simulink model "th4_general"  (R2023b)
settings: Solver=VariableStepAuto  StartTime=0.0  StopTime=1000  RelTol=1e-3
values from neighbouring files (symbols this model uses):
  A = 1.2    [part1_q4.m]
  battery_capacity = 20    [th4_init.m]
  Cd = 0.5    [part1_q4.m]
  f = 0.015    [part1_q4.m]    (also in th4_q19.m; th4_q19_claude.m)
  g = 9.81    [part1_q4.m]    (also in th4_q19.m; th4_q19_claude.m; th4_q19_create_road_grade.m = segments(i,3))
  m = 1250    [part1_q4.m]    (also in th4_q19_battery_pps.m = 1305.3)
  m_eqv = m + I_w_total/r^2 + I_e*(G*R)^2/r^2    (= 1305.28194444)    [part1_q4.m]    (also in th4_q19.m = 1305.3; th4_q19_claude.m = 1305.3)
  mu_driveline = 0.8    [th4_init.m]
  mu_generator = 0.9    [th4_init.m]
  R_w = 0.5    [th4_init.m]
  ro = 1.225    [part1_q4.m]
  SOC_init = 0.6    [th4_init.m]
  SOC_max = 0.95    [th4_init.m]
  SOC_min = 0.2    [th4_init.m]
libraries: simulink x2, simulink_extras x2, slpidlib x1
settings Model: Creator=yusufcagriogut  LastModifiedBy=yusufcagriogut

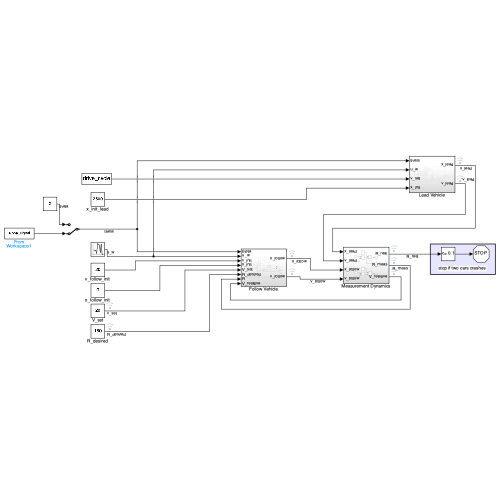
[thumbnail: Simulink's stored preview of the top-level diagram]
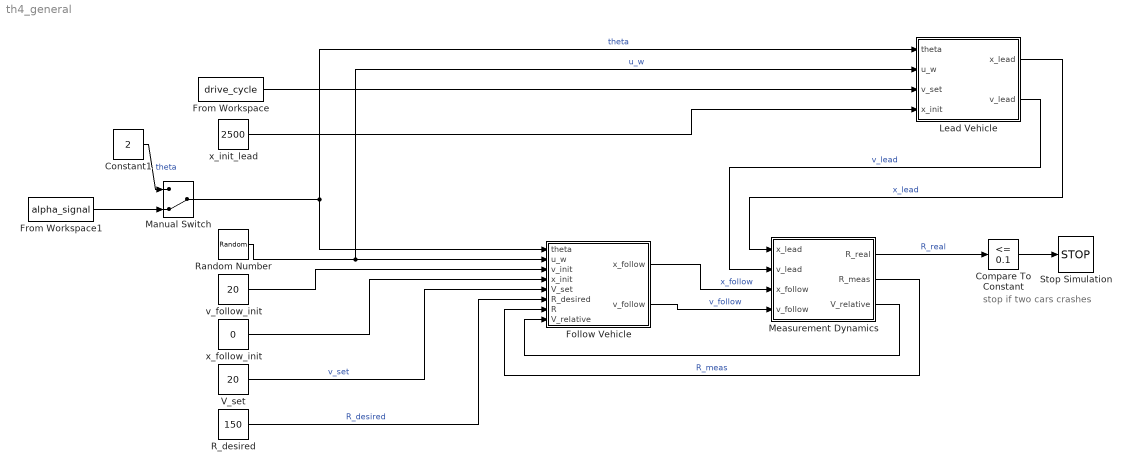
== system th4_general ==
  note: stop if two cars crashes
  Compare To Constant : simulink/Logic and Bit Operations/Compare To Constant  relop=<=  const=0.1  OutDataTypeStr=boolean
  Constant1 : Constant  Value=2
  Follow Vehicle : Subsystem
  From Workspace : FromWorkspace  VariableName=drive_cycle
  From Workspace1 : FromWorkspace  VariableName=alpha_signal
  Lead Vehicle : Subsystem
  Manual Switch : ManualSwitch  CurrentSetting=0
  Measurement Dynamics : Subsystem
  R_desired : Constant  Value=150
  Random Number : RandomNumber  Variance=2  SampleTime=2
  Stop Simulation : Stop
  V_set : Constant  Value=20
  v_follow_init : Constant  Value=20
  x_follow_init : Constant  Value=0
  x_init_lead : Constant  Value=2500
  wires:
  Lead Vehicle/2(v_lead) -> Measurement Dynamics/2(v_lead)  "v_lead"
  Lead Vehicle/1(x_lead) -> Measurement Dynamics/1(x_lead)  "x_lead"
  Measurement Dynamics/2(R_meas) -> Follow Vehicle/7(R)  "R_meas"
  Follow Vehicle/1(x_follow) -> Measurement Dynamics/3(x_follow)  "x_follow"
  Follow Vehicle/2(v_follow) -> Measurement Dynamics/4(v_follow)  "v_follow"
  Measurement Dynamics/3(V_relative) -> Follow Vehicle/8(V_relative)
  Manual Switch/1 -> Follow Vehicle/1(theta), Lead Vehicle/1(theta)  "theta"
  Random Number/1 -> Lead Vehicle/2(u_w), Follow Vehicle/2(u_w)  "u_w"
  From Workspace/1 -> Lead Vehicle/3(v_set)
  x_init_lead/1 -> Lead Vehicle/4(x_init)
  v_follow_init/1 -> Follow Vehicle/3(v_init)
  x_follow_init/1 -> Follow Vehicle/4(x_init)
  Measurement Dynamics/1(R_real) -> Compare To Constant/1  "R_real"
  V_set/1 -> Follow Vehicle/5(V_set)  "v_set"
  R_desired/1 -> Follow Vehicle/6(R_desired)  "R_desired"
  Compare To Constant/1 -> Stop Simulation/1
  Constant1/1 -> Manual Switch/1  "theta"
  From Workspace1/1 -> Manual Switch/2

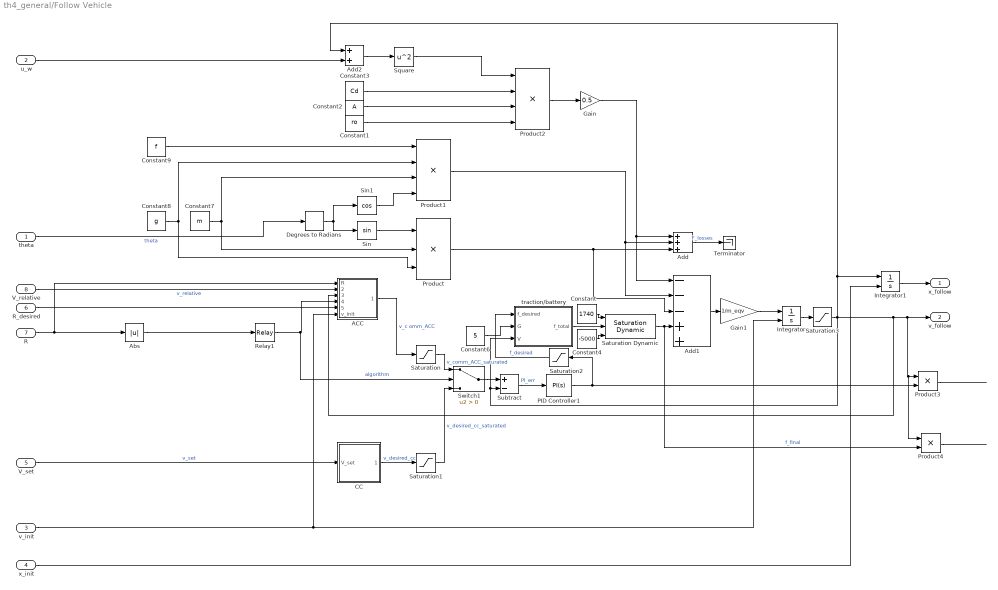
== system th4_general/Follow Vehicle ==
  theta : Inport
  u_w : Inport  Port=2
  v_init : Inport  Port=3
  x_init : Inport  Port=4
  V_set : Inport  Port=5
  R_desired : Inport  Port=6
  R : Inport  Port=7
  V_relative : Inport  Port=8
  ACC : Subsystem
  Abs : Abs  SaturateOnIntegerOverflow=off
  Add : Sum  Inputs=+++
  Add1 : Sum  Inputs=---++
  Add2 : Sum
  CC : Subsystem
  Constant : Constant  Value=1740
  Constant1 : Constant  Value=ro
  Constant2 : Constant  Value=A
  Constant3 : Constant  Value=Cd
  Constant4 : Constant  Value=-5000
  Constant6 : Constant  Value=5
  Constant7 : Constant  Value=m
  Constant8 : Constant  Value=g
  Constant9 : Constant  Value=f
  Degrees to Radians : simulink_extras/Transformations/Degrees to Radians
  Gain : Gain  Gain=0.5
  Gain1 : Gain  Gain=1/m_eqv
  Integrator : Integrator  InitialConditionSource=external  InitialCondition=33
  Integrator1 : Integrator  InitialConditionSource=external
  PID Controller1 : slpidlib/PID Controller  Controller=PI  Form=Parallel  TimeDomain=Continuous-time  UseExternalTs=off  SampleTime=-1  IntegratorMethod=Forward Euler  FilterMethod=Forward Euler  ControllerParametersSource=internal  P=600  I=50  UseKiTs=off  D=0  N=12.815158437423  UseFilter=on  TunerSelectOption=Transfer Function Based (PID Tuner App)  InitialConditionSource=internal  InitialConditionForIntegrator=0  InitialConditionForFilter=0  DifferentiatorICPrevScaledInput=0  ExternalReset=none  TrackingMode=off  Kt=1  LimitOutput=off  SatLimitsSource=internal  UpperSaturationLimit=inf  LowerSaturationLimit=-inf  LinearizeAsGain=on  AntiWindupMode=none  Kb=1  LimitIntegrator=off  UpperIntegratorSaturationLimit=inf  LowerIntegratorSaturationLimit=-inf  POutMin=[]  POutMax=[]  IOutMin=[]  IOutMax=[]  DOutMin=[]  DOutMax=[]  NOutMin=[]  NOutMax=[]  SumOutMin=[]  SumOutMax=[]  SaturationOutMin=[]  SaturationOutMax=[]  PParamMin=[]  PParamMax=[]  IParamMin=[]  IParamMax=[]  DParamMin=[]  DParamMax=[]  NParamMin=[]  NParamMax=[]  KbParamMin=[]  KbParamMax=[]  KtParamMin=[]  KtParamMax=[]  KbOutMin=[]  KbOutMax=[]  KtOutMin=[]  KtOutMax=[]  IntegratorOutMin=[]  IntegratorOutMax=[]  FilterOutMin=[]  FilterOutMax=[]  SumI1OutMin=[]  SumI1OutMax=[]  SumI2OutMin=[]  SumI2OutMax=[]  SumI3OutMin=[]  SumI3OutMax=[]  SumI4OutMin=[]  SumI4OutMax=[]  SumDOutMin=[]  SumDOutMax=[]  DifferentiatorOutMin=[]  DifferentiatorOutMax=[]  FilterDiffOutCoefMin=[]  FilterDiffOutCoefMax=[]  ReciprocalOutMin=[]  ReciprocalOutMax=[]  SumDenOutMin=[]  SumDenOutMax=[]  SumNumOutMin=[]  SumNumOutMax=[]  DivideOutMin=[]  DivideOutMax=[]  UdiffTsProdOutMin=[]  UdiffTsProdOutMax=[]  NTsProdOutMin=[]  NTsProdOutMax=[]  UintegralTsProdOutMin=[]  UintegralTsProdOutMax=[]  UngainTsProdOutMin=[]  UngainTsProdOutMax=[]  ClampingZeroOutDataTypeStr=Inherit: Inherit via back propagation  ClampingZeroOutMin=[]  ClampingZeroOutMax=[]  FilterDenConstantOutDataTypeStr=Inherit: Inherit via back propagation  FilterDenConstantOutMin=[]  FilterDenConstantOutMax=[]  PCopyOutDataTypeStr=Inherit: Inherit via back propagation  PCopyOutMin=[]  PCopyOutMax=[]  NCopyOutDataTypeStr=Inherit: Inherit via back propagation  NCopyOutMin=[]  NCopyOutMax=[]  IntegratorContinuousStateAttributes=''  IntegratorStateMustResolveToSignalObject=off  IntegratorRTWStateStorageClass=Auto  FilterContinuousStateAttributes=''  FilterStateMustResolveToSignalObject=off  FilterRTWStateStorageClass=Auto  ParallelPVariant=InternalParameters  IdealPVariant=Disabled  IVariant=InternalParameters  DVariant=Disabled  IntegratorVariant=Continuous  SatVariant=Disabled  AWVariant=Passthrough  PCopyVariant=Disabled  TRVariant=Disabled  FdbkBlocksVariant=Forward  IdealPFdbkVariant=Disabled  SatFdbkVariant=Disabled  DerivativeFilterVariant=Disabled  NVariant=Disabled  NCopyVariant=Disabled_SignalSpec  FilterICVariant=Disabled  IntegratorICVariant=InternalICs  ExternalResetVariant=Disabled  TRSumVariant=Passthrough  SumFdbkVariant=Disabled  SumVariant=Sum_PI  TsampFilterVariant=InternalTs  TsampNgainVariant=Passthrough  TsampIntegralVariant=Disabled_SignalSpec  ExternalSaturationOutDataTypeStr=Inherit: Same as second input
  Product : Product  Inputs=3
  Product1 : Product  Inputs=4
  Product2 : Product  Inputs=4
  Product3 : Product
  Product4 : Product
  Relay1 : Relay  OnSwitchValue=160  OffSwitchValue=140  OnOutputValue=0  OffOutputValue=1
  Saturation : Saturate  UpperLimit=50  LowerLimit=-50
  Saturation Dynamic : simulink/Discontinuities/Saturation Dynamic  OutMin=[]  OutMax=[]  OutDataTypeStr=Inherit: Same as second input  OutDataType=fixdt(1, 16)  OutScaling=2^-10  DoSatur=off
  Saturation1 : Saturate  UpperLimit=50  LowerLimit=0
  Saturation2 : Saturate  UpperLimit=1740  LowerLimit=-5000
  Saturation3 : Saturate  UpperLimit=120  LowerLimit=0
  Sin : Trigonometry
  Sin1 : Trigonometry  Operator=cos
  Square : Math  Operator=square
  Subtract : Sum  Inputs=+-
  Switch1 : Switch  Criteria=u2 > Threshold  SaturateOnIntegerOverflow=off  InputSameDT=off
  Terminator : Terminator
  traction/battery : Subsystem
  x_follow : Outport
  v_follow : Outport  Port=2
  wires:
  Integrator1/1 -> x_follow/1
  R/1 -> ACC/1(R), Abs/1
  Abs/1 -> Relay1/1
  Gain1/1 -> Integrator/1
  Add1/1 -> Gain1/1
  Product2/1 -> Gain/1
  Add2/1 -> Square/1
  Constant1/1 -> Product2/4
  Constant2/1 -> Product2/3
  Constant3/1 -> Product2/2
  u_w/1 -> Add2/2
  Square/1 -> Product2/1
  Integrator/1 -> Saturation3/1
  Gain/1 -> Add/1, Add1/1
  theta/1 -> Degrees to Radians/1  "theta"
  Sin/1 -> Product/1
  Product/1 -> Add1/3, Add/3
  Constant8/1 -> Product/3, Product1/2
  Sin1/1 -> Product1/4
  Constant7/1 -> Product/2, Product1/3
  Product1/1 -> Add1/2, Add/2
  Constant9/1 -> Product1/1
  Degrees to Radians/1 -> Sin/1, Sin1/1
  v_init/1 -> ACC/6(v_init), Integrator/2
  x_init/1 -> Integrator1/2
  V_relative/1 -> ACC/2(V_relative)  "v_relative"
  V_set/1 -> CC/1(V_set)  "v_set"
  Saturation/1 -> Switch1/1  "v_comm_ACC_saturated"
  ACC/1(v_desired) -> Saturation/1  "v_c omm_ACC"
  Switch1/1 -> Subtract/1
  CC/1(V_desired) -> Saturation1/1  "v_desired_cc"
  Saturation1/1 -> Switch1/3  "v_desired_cc_saturated"
  R_desired/1 -> ACC/5(R_desired)
  Saturation Dynamic/1 -> Product4/2, Add1/4  "f_final"
  Constant/1 -> Saturation Dynamic/1
  Constant4/1 -> Saturation Dynamic/3
  PID Controller1/1 -> Saturation2/1, Product3/2
  Subtract/1 -> PID Controller1/1  "PI_err"
  Relay1/1 -> ACC/4(active), Switch1/2  "algorithm"
  Product3/1 -> ?
  Product4/1 -> ?
  Constant6/1 -> traction/battery/2(G)
  Saturation2/1 -> traction/battery/1(f_desired)  "f_desired"
  Saturation3/1 -> Add2/1, Integrator1/1, traction/battery/3(V), Subtract/2, ACC/3(V_follow), Product4/1, Product3/1, v_follow/1
  traction/battery/1(f_total) -> Saturation Dynamic/2
  Add/1 -> Terminator/1  "F_losses"

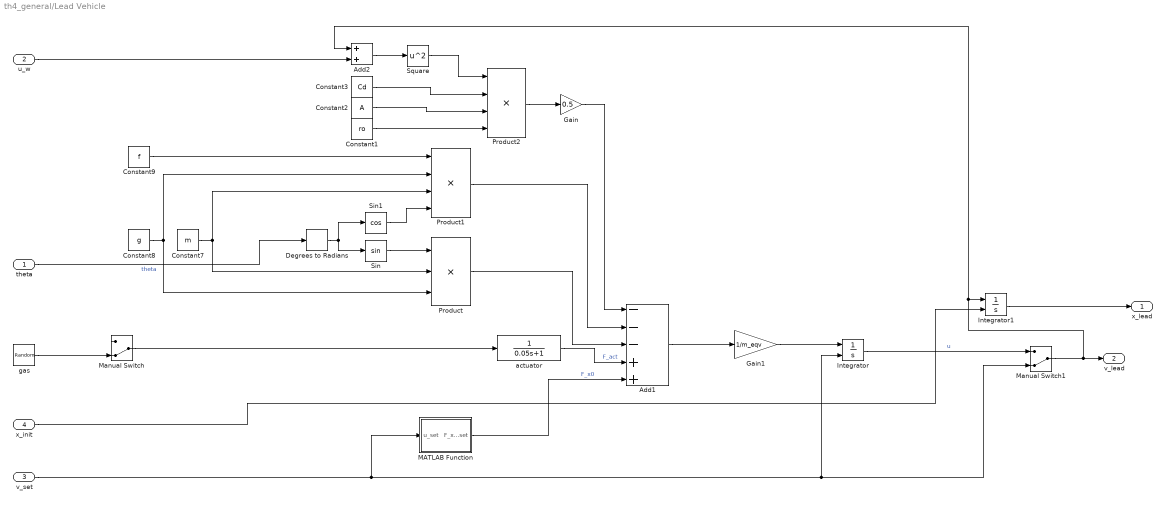
== system th4_general/Lead Vehicle ==
  theta : Inport
  u_w : Inport  Port=2
  v_set : Inport  Port=3
  x_init : Inport  Port=4
  Add1 : Sum  Inputs=---++
  Add2 : Sum
  Constant1 : Constant  Value=ro
  Constant2 : Constant  Value=A
  Constant3 : Constant  Value=Cd
  Constant7 : Constant  Value=m
  Constant8 : Constant  Value=g
  Constant9 : Constant  Value=f
  Degrees to Radians : simulink_extras/Transformations/Degrees to Radians
  Gain : Gain  Gain=0.5
  Gain1 : Gain  Gain=1/m_eqv
  Integrator : Integrator  InitialConditionSource=external  InitialCondition=33
  Integrator1 : Integrator  InitialConditionSource=external
  MATLAB Function : MATLAB Function  TreatAsAtomicUnit=on
  Manual Switch : ManualSwitch  CurrentSetting=0
  Manual Switch1 : ManualSwitch  CurrentSetting=0
  Product : Product  Inputs=3
  Product1 : Product  Inputs=4
  Product2 : Product  Inputs=4
  Sin : Trigonometry
  Sin1 : Trigonometry  Operator=cos
  Square : Math  Operator=square
  actuator : TransferFcn  Denominator=[0.05 1]
  gas : RandomNumber  Variance=0  SampleTime=2
  x_lead : Outport
  v_lead : Outport  Port=2
  wires:
  Integrator1/1 -> x_lead/1
  Gain1/1 -> Integrator/1
  Add1/1 -> Gain1/1
  v_set/1 -> Manual Switch1/2, Integrator/2, MATLAB Function/1(u_set)
  actuator/1 -> Add1/4  "F_act"
  Product2/1 -> Gain/1
  Add2/1 -> Square/1
  Constant1/1 -> Product2/4
  Constant2/1 -> Product2/3
  Constant3/1 -> Product2/2
  u_w/1 -> Add2/2
  Square/1 -> Product2/1
  Integrator/1 -> Manual Switch1/1  "u"
  Gain/1 -> Add1/1
  theta/1 -> Degrees to Radians/1  "theta"
  Sin/1 -> Product/1
  Product/1 -> Add1/3
  Constant8/1 -> Product/3, Product1/2
  Sin1/1 -> Product1/4
  Constant7/1 -> Product/2, Product1/3
  Product1/1 -> Add1/2
  Constant9/1 -> Product1/1
  Degrees to Radians/1 -> Sin/1, Sin1/1
  x_init/1 -> Integrator1/2
  MATLAB Function/1(F_x0_set) -> Add1/5  "F_x0"
  Manual Switch/1 -> actuator/1
  gas/1 -> Manual Switch/2
  Manual Switch1/1 -> Add2/1, Integrator1/1, v_lead/1

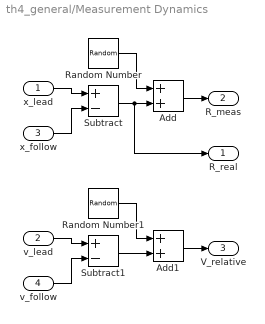
== system th4_general/Measurement Dynamics ==
  x_lead : Inport
  v_lead : Inport  Port=2
  x_follow : Inport  Port=3
  v_follow : Inport  Port=4
  Add : Sum
  Add1 : Sum
  Random Number : RandomNumber  Variance=0.2  SampleTime=0.1
  Random Number1 : RandomNumber  Variance=0.1  SampleTime=0.1
  Subtract : Sum  Inputs=+-
  Subtract1 : Sum  Inputs=+-
  R_real : Outport
  R_meas : Outport  Port=2
  V_relative : Outport  Port=3
  wires:
  Add/1 -> R_meas/1
  x_lead/1 -> Subtract/1
  x_follow/1 -> Subtract/2
  Subtract/1 -> R_real/1, Add/2
  Random Number/1 -> Add/1
  Add1/1 -> V_relative/1
  Subtract1/1 -> Add1/2
  Random Number1/1 -> Add1/1
  v_follow/1 -> Subtract1/2
  v_lead/1 -> Subtract1/1

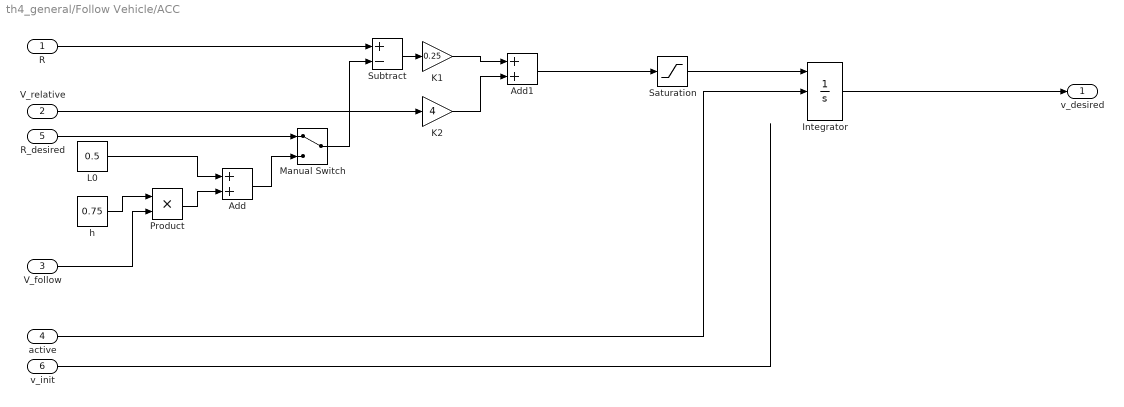
== system th4_general/Follow Vehicle/ACC ==
  R : Inport
  V_relative : Inport  Port=2
  V_follow : Inport  Port=3
  active : Inport  Port=4
  R_desired : Inport  Port=5
  v_init : Inport  Port=6
  Add : Sum
  Add1 : Sum
  Integrator : Integrator  ExternalReset=rising  InitialConditionSource=external  LimitOutput=on  UpperSaturationLimit=50  LowerSaturationLimit=0
  K1 : Gain  Gain=0.25
  K2 : Gain  Gain=4
  L0 : Constant  Value=0.5
  Manual Switch : ManualSwitch
  Product : Product
  Saturation : Saturate  UpperLimit=2.5  LowerLimit=-1
  Subtract : Sum  Inputs=+-
  h : Constant  Value=0.75
  v_desired : Outport
  wires:
  R/1 -> Subtract/1
  h/1 -> Product/1
  V_follow/1 -> Product/2
  L0/1 -> Add/1
  Product/1 -> Add/2
  Subtract/1 -> K1/1
  V_relative/1 -> K2/1
  K1/1 -> Add1/1
  Add1/1 -> Saturation/1
  active/1 -> Integrator/2
  R_desired/1 -> Manual Switch/1
  K2/1 -> Add1/2
  v_init/1 -> ?
  Add/1 -> Manual Switch/2
  Manual Switch/1 -> Subtract/2
  Saturation/1 -> Integrator/1
  Integrator/1 -> v_desired/1

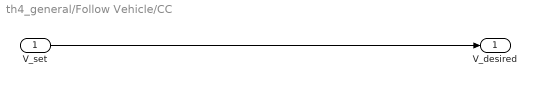
== system th4_general/Follow Vehicle/CC ==
  V_set : Inport
  V_desired : Outport
  wires:
  V_set/1 -> V_desired/1

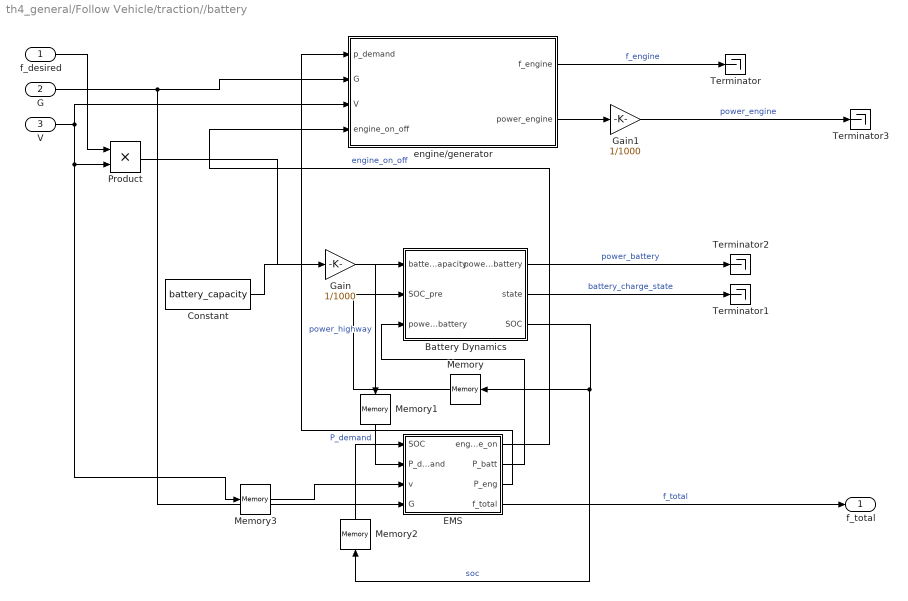
== system th4_general/Follow Vehicle/traction//battery ==
  f_desired : Inport
  G : Inport  Port=2
  V : Inport  Port=3
  Battery Dynamics : MATLAB Function  TreatAsAtomicUnit=on
  Constant : Constant  Value=battery_capacity
  EMS : Subsystem
  Gain : Gain  Gain=1/1000
  Gain1 : Gain  Gain=1/1000
  Memory : Memory  InitialCondition=SOC_init
  Memory1 : Memory
  Memory2 : Memory  InitialCondition=SOC_init
  Memory3 : Memory  InitialCondition=20
  Product : Product
  Terminator{,1..3} (4 alike) : Terminator
  engine/generator : Subsystem
  f_total : Outport
  wires:
  f_desired/1 -> Product/1
  G/1 -> engine/generator/2(G), EMS/4(G)
  V/1 -> Memory3/1, Product/2, engine/generator/3(V)
  engine/generator/2(power_engine) -> Gain1/1
  Battery Dynamics/3(SOC) -> Memory2/1, Memory/1  "soc"
  Product/1 -> Gain/1
  Memory/1 -> Battery Dynamics/2(SOC_pre)
  Constant/1 -> Battery Dynamics/1(battery_capacity)
  engine/generator/1(f_engine) -> Terminator/1  "f_engine"
  Battery Dynamics/2(state) -> Terminator1/1  "battery_charge_state"
  Battery Dynamics/1(power_battery) -> Terminator2/1  "power_battery"
  Gain/1 -> Memory1/1  "power_highway"
  Gain1/1 -> Terminator3/1  "power_engine"
  EMS/1(engine_on) -> engine/generator/4(engine_on_off)  "engine_on_off"
  EMS/3(P_eng) -> engine/generator/1(p_demand)
  EMS/2(P_batt) -> Battery Dynamics/3("power_battery ")
  Memory1/1 -> EMS/2(P_demand)  "P_demand"
  Memory2/1 -> EMS/1(SOC)
  Memory3/1 -> EMS/3(v)
  EMS/4(f_total) -> f_total/1  "f_total"

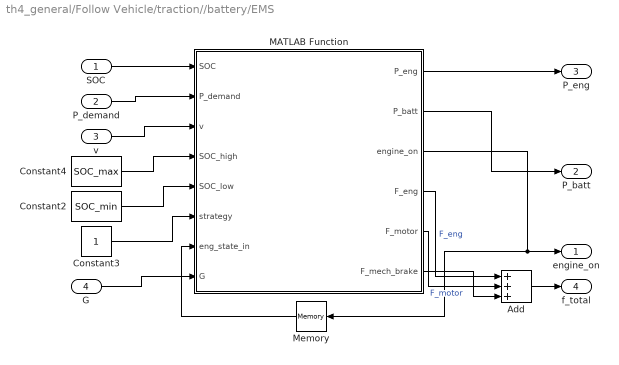
== system th4_general/Follow Vehicle/traction//battery/EMS ==
  SOC : Inport
  P_demand : Inport  Port=2
  v : Inport  Port=3
  G : Inport  Port=4
  Add : Sum  Inputs=+++
  Constant2 : Constant  Value=SOC_min
  Constant3 : Constant
  Constant4 : Constant  Value=SOC_max
  MATLAB Function : MATLAB Function  TreatAsAtomicUnit=on
  Memory : Memory  InitialCondition=1
  engine_on : Outport
  P_batt : Outport  Port=2
  P_eng : Outport  Port=3
  f_total : Outport  Port=4
  wires:
  Constant3/1 -> MATLAB Function/6(strategy)
  SOC/1 -> MATLAB Function/1(SOC)
  Constant2/1 -> MATLAB Function/5(SOC_low)
  Constant4/1 -> MATLAB Function/4(SOC_high)
  P_demand/1 -> MATLAB Function/2(P_demand)
  v/1 -> MATLAB Function/3(v)
  MATLAB Function/2(P_batt) -> P_batt/1
  MATLAB Function/1(P_eng) -> P_eng/1
  MATLAB Function/3(engine_on) -> Memory/1, engine_on/1
  Memory/1 -> MATLAB Function/7(eng_state_in)
  G/1 -> MATLAB Function/8(G)
  MATLAB Function/4(F_eng) -> Add/1  "F_eng"
  MATLAB Function/5(F_motor) -> Add/2  "F_motor"
  Add/1 -> f_total/1
  MATLAB Function/6(F_mech_brake) -> Add/3

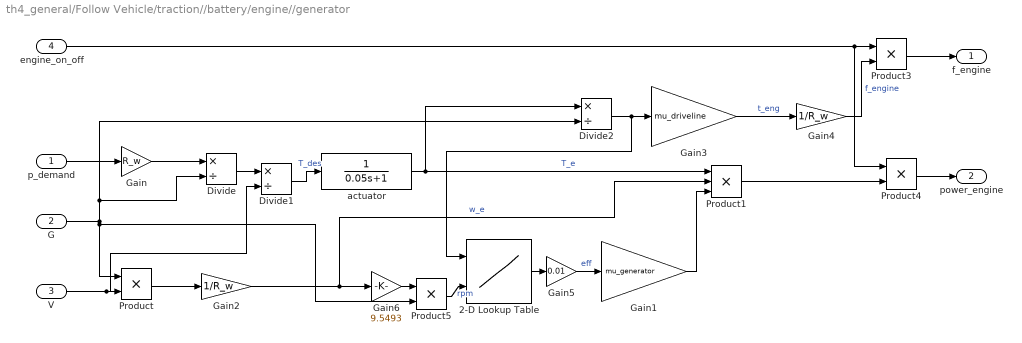
== system th4_general/Follow Vehicle/traction//battery/engine//generator ==
  p_demand : Inport
  G : Inport  Port=2
  V : Inport  Port=3
  engine_on_off : Inport  Port=4
  2-D Lookup Table : Lookup_n-D  BreakpointsForDimension1=[0, 20, 40, 60, 80, 100, 120, 140, 160, 174]  BreakpointsForDimension2=[800, 1200, 1600, 2000, 2500, 3000, 3500, 4000, 4500, 5000, 5500, 6000]  Table=[3,4,5,5.50000000000000,6,6,5.50000000000000,5,4.50000000000000,4,3.50000000000000,3;8,11,14,16,17,17.5000000000000,17,16,15,13.5000000000000,11.5000000000000,9;13,18,22,25,27,28,27.5000000000000,26.5000000000000,25,22.5000000000000,19.5000000000000,15;17,22,27,30,32,33,32.5000000000000,31.5000000000000,30,27.5000000000000,24,19;20,26,30.5000000000000,33.5000000000000,35,35.5000000000000,35,34,32.5000000000000,30,26.5000000000000,21.5000000000000;22.5000000000000,28.5000000000000,32.5000000000000,35,36.5000000000000,37,36.5000000000000,35.5000000000000,34,31.5000000000000,28,23;24,30,33.5000000000000,35.5000000000000,37,37.5000000000000,37,36,34.5000000000000,32,28.5000000000000,23.5000000000000;24.5000000000000,30.5000000000000,34,36,37.5000000000000,38,37.5000000000000,36.5000000000000,35,32.5000000000000,29,24;24,30,33.5000000000000,36,37.5000000000000,38,37.5000000000000,36.5000000000000,35,32.5000000000000,29,24;23,29.5000000000000,33,35.5000000000000,37,37.5000000000000,37,36,34.5000000000000,32,28.5000000000000,23.5000000000000]  InternalRulePriority=Speed  RndMeth=Simplest
      settings: InputPortMap=u0,u1
  Divide : Product  Inputs=*/
  Divide1 : Product  Inputs=*/
  Divide2 : Product  Inputs=*/
  Gain : Gain  Gain=R_w
  Gain1 : Gain  Gain=mu_generator
  Gain2 : Gain  Gain=1/R_w
  Gain3 : Gain  Gain=mu_driveline
  Gain4 : Gain  Gain=1/R_w
  Gain5 : Gain  Gain=0.01
  Gain6 : Gain  Gain=9.5493
  Product{,3..5} (4 alike) : Product
  Product1 : Product  Inputs=3
  actuator : TransferFcn  Denominator=[0.05 1]
  f_engine : Outport
  power_engine : Outport  Port=2
  wires:
  Gain4/1 -> Product3/2  "f_engine"
  Divide2/1 -> 2-D Lookup Table/1, Gain3/1
  Gain/1 -> Divide/1
  Gain3/1 -> Gain4/1  "t_eng"
  p_demand/1 -> Gain/1
  Product/1 -> Gain2/1
  2-D Lookup Table/1 -> Gain5/1
  G/1 -> Product5/2, Product/1, Divide2/2, Divide/2
  Divide/1 -> Divide1/1
  actuator/1 -> Divide2/1, Product1/1  "T_e"
  V/1 -> Divide1/2, Product/2
  Gain2/1 -> Gain6/1, Product1/2  "w_e"
  Gain5/1 -> Gain1/1  "eff"
  Gain6/1 -> Product5/1
  engine_on_off/1 -> Product4/1, Product3/1
  Product3/1 -> f_engine/1
  Product1/1 -> Product4/2
  Product4/1 -> power_engine/1
  Divide1/1 -> actuator/1  "T_des"
  Product5/1 -> 2-D Lookup Table/2  "rpm"
  Gain1/1 -> Product1/3

== matlab function th4_general/Lead Vehicle/MATLAB Function ==
  data: u_set input; F_x0_set output
function F_x0_set = fcn(u_set)
m = 1250;
ro = 1.225;
A = 1.2;
Cd = 0.5;
f = 0.015;
R = 3;
I_e = 0.15;
r = 0.3;
I_w = 1.0;
u_0 = 40;
u_w = 2;
g = 9.81;
theta_0 = 0;
F_x0_set = m*g*sin(theta_0) + f*m*g*cos(theta_0) + ...
    0.5*ro*A*Cd*(u_set+u_w)^2;
end

== matlab function th4_general/Follow Vehicle/traction//battery/Battery Dynamics ==
  data: power_battery output; battery_capacity input; SOC_pre input; state output; SOC output; power_battery input
function [power_battery, state,SOC] = fcn(battery_capacity, SOC_pre, power_battery)
if power_battery>0
    state = 0; % supply
else
    state = 1; % charging
end
SOC = SOC_pre - power_battery * 1 / 3600 / 0.92 / battery_capacity;
if SOC<0
    SOC = 0;
elseif SOC>1
    SOC = 1;
end
end

== matlab function th4_general/Follow Vehicle/traction//battery/EMS/MATLAB Function ==
  data: SOC input; P_eng output; P_demand input; v input; SOC_high input; SOC_low input; strategy input; P_batt output; engine_on output; eng_state_in input; G input; F_eng output; F_motor output; F_mech_brake output
function [P_eng, P_batt, engine_on, F_eng, F_motor,F_mech_brake] = EMS(SOC, P_demand, v, SOC_high, SOC_low, strategy, eng_state_in, G)

%% Parameters
P_eng_max   = 60.0;
P_eng_opt   = 20.0;
v_min       = 1.0;
P_regen_max = 30.0;
r_wheel     = 0.5;
T_eng_max   = 174;
P_motor_kW  = 69.0;
Vb          = 40/3.6;
F_motor_max = (P_motor_kW * 1000) / Vb;

%% Defaults
P_eng     = 0;
P_batt    = 0;
engine_on = 0;
P_mech_brake = 0;
%% ---- Decision logic (no early returns) ----
if P_demand < 0
    if SOC >= SOC_high
        P_batt       = 0;
        P_mech_brake = P_demand;        % all braking is mechanical
    else
        P_batt       = max(P_demand, -P_regen_max);
        P_mech_brake = P_demand - P_batt;  % remainder after regen
    end
    P_eng     = 0;
    engine_on = 0;

elseif v < v_min
    %% Standstill
    P_eng     = 0;
    P_batt    = P_demand;
    engine_on = 0;

elseif strategy == 1
    %% On-Off
    if SOC <= SOC_low
        P_eng     = min(P_eng_opt, P_eng_max);
        P_batt    = P_demand - P_eng;
        engine_on = 1;
    elseif SOC >= SOC_high
        P_eng     = 0;
        P_batt    = P_demand;
        engine_on = 0;
    else
        if eng_state_in == 1
            P_eng  = min(P_eng_opt, P_eng_max);
            P_batt = P_demand - P_eng;
        else
            P_eng  = 0;
            P_batt = P_demand;
        end
        engine_on = eng_state_in;
    end

elseif strategy == 2
    %% Max SOC
    if SOC >= SOC_high
        % Battery full — engine covers only exact demand
        P_eng     = min(P_demand, P_eng_max);
        P_batt    = P_demand - P_eng;
        engine_on = 1;

    elseif SOC < SOC_low
        % Battery critically low — engine at max to recharge fast
        P_eng     = P_eng_max;
        P_batt    = P_demand - P_eng;
        engine_on = 1;

    else
        % Normal band — engine ALWAYS runs at optimal point
        % regardless of P_demand, to proactively charge battery
        P_eng     = P_eng_opt;           % <-- was: min(P_demand, P_eng_opt)
        P_batt    = P_demand - P_eng;    % will be negative = charging
        engine_on = 1;                   % <-- was: conditional on P_eng > 0
    end

else
    P_eng     = 0;
    P_batt    = P_demand;
    engine_on = 0;
end

%% ---- Safety clamps ----
P_eng  = max(0, min(P_eng, P_eng_max));
P_batt = max(-P_regen_max, P_batt);

%% ---- Force conversion (runs for ALL cases now) ----
% Mechanical brake force (always negative or zero)
v_safe       = max(v, v_min);
F_mech_brake = (P_mech_brake * 1000) / v_safe;
v_safe  = max(v, v_min);

F_eng   = (P_eng  * 1000) / v_safe;
F_motor = (P_batt * 1000) / v_safe;

F_eng   = min(F_eng,  T_eng_max * G / r_wheel);
F_motor = min(abs(F_motor), F_motor_max) * sign(F_motor);
